simulink model "TRAS_identification"  (R2013a)
settings: Solver=ode5  SolverMode=SingleTasking  StartTime=0.0  StopTime=stop_time  FixedStep=sampling_time  RelTol=1e-3  AbsTol=1e-6
undefined symbols (not defined in the file): rtdac4pcibaseaddress
libraries: simulink x2
settings Model: SimulationMode=external  ExtModeTrigDuration=12000  ExtModeTrigLevel=0.400000  Creator=jims  LastModifiedBy=calc2
settings DataIOCC: ExternalInput=[]  InitialState=[]  LimitDataPoints=off  MaxDataPoints=5000  SignalLoggingSaveFormat=ModelDataLogs  SaveOutput=off  SaveTime=off  SignalLoggingName=sigsOut
settings OptimizationCC: BooleanDataType=off  ExpressionDepthLimit=2147483647  InitFltsAndDblsToZero=on
settings DebuggingCC: SaveWithParameterizedLinksMsg=none  MergeDetectMultiDrivingBlocksExec=error  SolverPrmCheckMsg=none  MultiTaskDSMMsg=warning  MultiTaskCondExecSysMsg=none  IntegerOverflowMsg=none  FcnCallInpInsideContextMsg=EnableAllAsWarning  StrictBusMsg=None
settings HardwareCC: TargetEndianess=LittleEndian  TargetHWDeviceType=MATLAB Host
settings RTWCC: SystemTargetFile=rtwin.tlc  TemplateMakefile=rtwin.tmf  Description=Real-Time Windows Target  ProcessScript=rtwin_make_rtw_hook  IncludeERTFirstTime=on
settings RTWinTargetCC: TargetFcnLib=ansi_tfl_tmw.mat  TargetLibSuffix=_rtwin.lib  TargetPreCompLibLocation=C:\Program Files\MATLAB\R2013a\toolbox\rtw\targets\rtwin\lib\win32  CodeReplacementLibrary=ANSI_C  ModelReferenceCompliant=off  CompOptLevelCompliant=off  RTWinDir=C:/PROGRA~1/MATLAB/R2013a/toolbox/rtw/targets/rtwin  TargetArch=win32

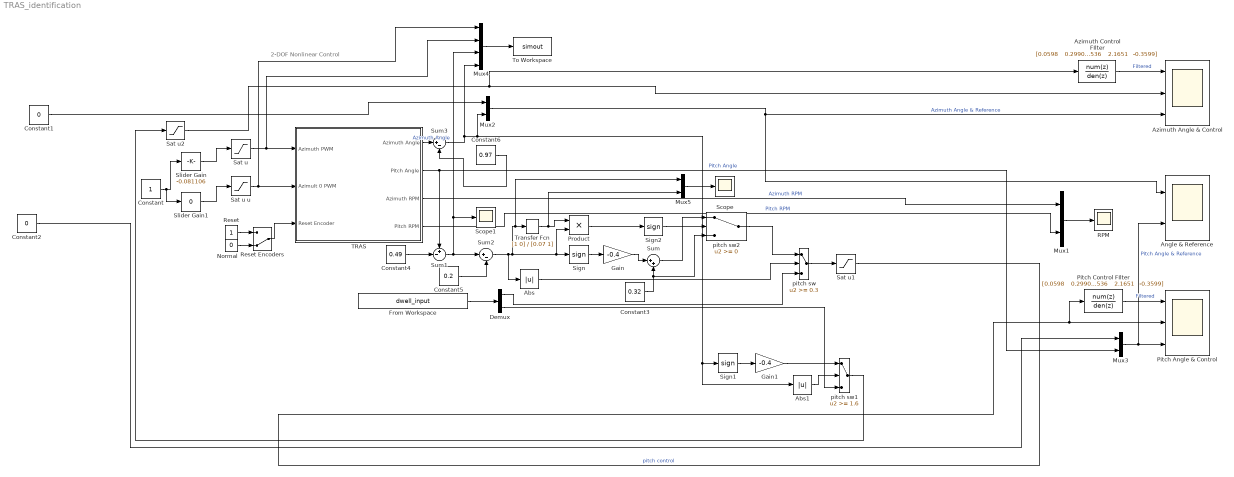
== system TRAS_identification ==
  note: 2-DOF Nonlinear Control
  Abs : Abs
  Abs1 : Abs
  Angle & Reference : Scope  NumInputPorts=2
      settings: TimeRange=90  YMin=-1~-0.5  YMax=1~0.4  SaveName=AngleReference_  MaxDataPoints=12000
  Azimuth Angle & Control : Scope  NumInputPorts=3
      settings: TimeRange=90  YMin=-0.4~-0.5~-1  YMax=-0.225~0.5~1  SaveName=AngleCtrl_  MaxDataPoints=12000
  Azimuth Control FIlter : DiscreteTransferFcn  Numerator="[0.0598    0.2990    0.5980    0.5980    0.2990    0.0598] * 1e-3"  Denominator="[1.0000   -3.9845    6.4349   -5.2536    2.1651   -0.3599]"  SampleTime=0.01
  Constant : Constant
  Constant1 : Constant  Value=0
  Constant2 : Constant  Value=0
  Constant3 : Constant  Value=0.32
  Constant4 : Constant  Value=0.49
  Constant5 : Constant  Value=0.2
  Constant6 : Constant  Value=0.97
  Demux : Demux  Outputs=2
  From Workspace : FromWorkspace  VariableName=dwell_input
  Gain : Gain  Gain=-0.4
  Gain1 : Gain  Gain=-0.4
  Mux{1..3,5} (4 alike) : Mux  Inputs=2
  Mux4 : Mux
  Normal : Constant  Value=0
  Pitch Angle & Control : Scope  NumInputPorts=3
      settings: TimeRange=90  YMin=2.77556e-17~-0.1~-0.5  YMax=0.75~0.9~0.35  SaveName=AngleCtrl1_  MaxDataPoints=12000
  Pitch Control FIlter : DiscreteTransferFcn  Numerator="[0.0598    0.2990    0.5980    0.5980    0.2990    0.0598] * 1e-3"  Denominator="[1.0000   -3.9845    6.4349   -5.2536    2.1651   -0.3599]"  SampleTime=0.01
  Product : Product
  RPM : Scope
      settings: TimeRange=90  YMin=-6000  YMax=7000  SaveName=RPM_  MaxDataPoints=12000
  Reset : Constant
  Reset Encoders : ManualSwitch  CurrentSetting=0
  Sat u : Saturate  UpperLimit=1  LowerLimit=-1
  Sat u u : Saturate  UpperLimit=1  LowerLimit=-1
  Sat u1 : Saturate  UpperLimit=1  LowerLimit=-1
  Sat u2 : Saturate  UpperLimit=1  LowerLimit=-1
  Scope : Scope
      settings: YMin=-2  YMax=2.25
  Scope1 : Scope
  Sign : Signum
  Sign1 : Signum
  Sign2 : Signum
  Slider Gain : simulink/Math Operations/Slider Gain  low=-1  gain=-0.081106  high=1
  Slider Gain1 : simulink/Math Operations/Slider Gain  low=-1  gain=0  high=1
  Sum : Sum  Inputs=|++
  Sum1 : Sum  Inputs=+-|
  Sum2 : Sum  Inputs=|+-
  Sum3 : Sum  Inputs=|+-
  TRAS : Subsystem  mask{BaseAddress=rtdac4pcibaseaddress, T0=0.01}
      mask prompts: BaseAddress "Base Address:"; T0 "Sampling Period:"
      mask Display: image(imread('TRAS.JPG'))
  To Workspace : ToWorkspace  VariableName=simout  SampleTime=-1  SaveFormat=Structure With Time
  Transfer Fcn : TransferFcn  Numerator=[1 0]  Denominator=[0.07 1]
  pitch sw : Switch  Threshold=0.3
  pitch sw1 : Switch  Threshold=1.6
  pitch sw2 : Switch
  wires:
  Pitch Control FIlter/1 -> Pitch Angle & Control/1  "Filtered"
  Mux3/1 -> Pitch Angle & Control/3, Angle & Reference/2  "Pitch Angle & Reference"
  TRAS/2(Pitch Angle) -> Sum1/1, Mux3/2  "Pitch Angle"
  Mux1/1 -> RPM/1
  Sat u2/1 -> Azimuth Angle & Control/2, Azimuth Control FIlter/1
  Sat u1/1 -> Pitch Angle & Control/2, Pitch Control FIlter/1  "pitch control"
  Azimuth Control FIlter/1 -> Azimuth Angle & Control/1  "Filtered"
  Mux2/1 -> Azimuth Angle & Control/3, Angle & Reference/1  "Azimuth Angle & Reference"
  Reset Encoders/1 -> TRAS/3(Reset Encoder)
  Reset/1 -> Reset Encoders/1
  Normal/1 -> Reset Encoders/2
  TRAS/4(Pitch RPM) -> Mux1/2  "Pitch RPM"
  TRAS/3(Azimuth RPM) -> Mux1/1  "Azimuth RPM"
  TRAS/1(Azimuth Angle) -> Sum3/1  "Azimuth Angle"
  Constant1/1 -> Mux2/1
  Constant2/1 -> Mux3/1
  From Workspace/1 -> Demux/1
  Mux4/1 -> To Workspace/1
  Sign/1 -> Gain/1
  Sum1/1 -> Scope1/1, Mux4/3, Sum2/1
  Constant4/1 -> Sum1/2
  Abs/1 -> pitch sw/2
  Demux/1 -> pitch sw/3
  pitch sw/1 -> Sat u1/1
  Gain1/1 -> pitch sw1/1
  Sign1/1 -> Gain1/1
  Abs1/1 -> pitch sw1/2
  Demux/2 -> pitch sw1/3
  pitch sw1/1 -> Sat u2/1
  Constant5/1 -> Sum2/2
  Sum2/1 -> Abs/1, Mux5/1, Transfer Fcn/1, Product/2, Sign/1
  Sum3/1 -> Mux4/4, Mux2/2, Abs1/1, Sign1/1
  Constant6/1 -> Sum3/2
  Product/1 -> Sign2/1
  Transfer Fcn/1 -> Mux5/2, Product/1
  Sign2/1 -> pitch sw2/2
  Gain/1 -> Sum/1
  Constant3/1 -> pitch sw2/3, Sum/2
  Sum/1 -> pitch sw2/1
  pitch sw2/1 -> pitch sw/1
  Mux5/1 -> Scope/1
  Sat u/1 -> Mux4/2, TRAS/1(Azimuth PWM)
  Sat u u/1 -> Mux4/1, TRAS/2(Azimult 0 PWM)
  Constant/1 -> Slider Gain1/1, Slider Gain/1
  Slider Gain/1 -> Sat u/1
  Slider Gain1/1 -> Sat u u/1

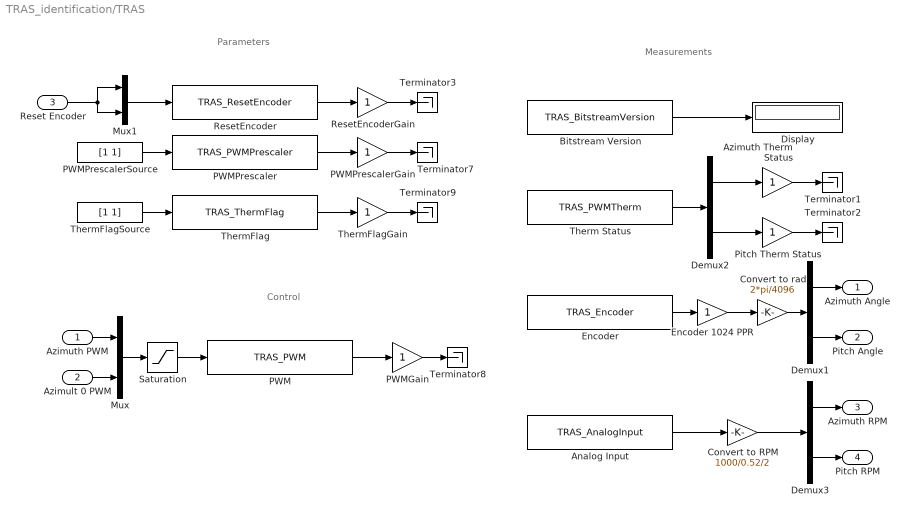
== system TRAS_identification/TRAS ==
  note: Parameters
  note: Control
  note: Measurements
  Azimuth PWM : Inport
  Azimult 0 PWM : Inport  Port=2
  Reset Encoder : Inport  Port=3
  Analog Input : S-Function  FunctionName=TRAS_AnalogInput  Parameters=BaseAddress, [1 0], [1 1], T0  EnableBusSupport=off
  Azimuth Therm Status : Gain  SaturateOnIntegerOverflow=on  OutDataTypeStr=Inherit: Same as input  ParamDataTypeStr=Inherit: Same as input
  Bitstream Version : S-Function  FunctionName=TRAS_BitstreamVersion  Parameters=BaseAddress, T0  EnableBusSupport=off
  Convert to RPM : Gain  Gain=1000/0.52/2  SaturateOnIntegerOverflow=on  OutDataTypeStr=Inherit: Same as input  ParamDataTypeStr=Inherit: Same as input
  Convert to rad : Gain  Gain=2*pi/4096  SaturateOnIntegerOverflow=on  OutDataTypeStr=Inherit: Same as input  ParamDataTypeStr=Inherit: Same as input
  Demux1 : Demux  Outputs=2
  Demux2 : Demux  Outputs=2
  Demux3 : Demux  Outputs=2
  Display : Display
  Encoder : S-Function  FunctionName=TRAS_Encoder  Parameters=BaseAddress, T0  EnableBusSupport=off
  Encoder 1024 PPR : Gain  SaturateOnIntegerOverflow=on  OutDataTypeStr=Inherit: Same as input  ParamDataTypeStr=Inherit: Same as input
  Mux : Mux  Inputs=2
  Mux1 : Mux  Inputs=2
  PWM : S-Function  FunctionName=TRAS_PWM  Parameters=BaseAddress, T0  EnableBusSupport=off
  PWMGain : Gain  SaturateOnIntegerOverflow=on  OutDataTypeStr=Inherit: Same as input  ParamDataTypeStr=Inherit: Same as input
  PWMPrescaler : S-Function  FunctionName=TRAS_PWMPrescaler  Parameters=BaseAddress, T0  EnableBusSupport=off
  PWMPrescalerGain : Gain  SaturateOnIntegerOverflow=on  OutDataTypeStr=Inherit: Same as input  ParamDataTypeStr=Inherit: Same as input
  PWMPrescalerSource : Constant  Value=[1 1]
  Pitch Therm Status : Gain  SaturateOnIntegerOverflow=on  OutDataTypeStr=Inherit: Same as input  ParamDataTypeStr=Inherit: Same as input
  ResetEncoder : S-Function  FunctionName=TRAS_ResetEncoder  Parameters=BaseAddress, T0  EnableBusSupport=off
  ResetEncoderGain : Gain  SaturateOnIntegerOverflow=on  OutDataTypeStr=Inherit: Same as input  ParamDataTypeStr=Inherit: Same as input
  Saturation : Saturate  UpperLimit=1  LowerLimit=-1
  Terminator{1..3,7..9} (6 alike) : Terminator
  Therm Status : S-Function  FunctionName=TRAS_PWMTherm  Parameters=BaseAddress, T0  EnableBusSupport=off
  "ThermFlag " : S-Function  FunctionName=TRAS_ThermFlag  Parameters=BaseAddress, T0  EnableBusSupport=off
  ThermFlagGain : Gain  SaturateOnIntegerOverflow=on  OutDataTypeStr=Inherit: Same as input  ParamDataTypeStr=Inherit: Same as input
  ThermFlagSource : Constant  Value=[1 1]
  Azimuth Angle : Outport  InitialOutput=0
  Pitch Angle : Outport  Port=2  InitialOutput=0
  Azimuth RPM : Outport  Port=3  InitialOutput=0
  Pitch RPM : Outport  Port=4  InitialOutput=0
  wires:
  Encoder 1024 PPR/1 -> Convert to rad/1
  Encoder/1 -> Encoder 1024 PPR/1
  Saturation/1 -> PWM/1
  Mux/1 -> Saturation/1
  PWM/1 -> PWMGain/1
  PWMGain/1 -> Terminator8/1
  ResetEncoder/1 -> ResetEncoderGain/1
  PWMPrescaler/1 -> PWMPrescalerGain/1
  Mux1/1 -> ResetEncoder/1
  PWMPrescalerSource/1 -> PWMPrescaler/1
  ResetEncoderGain/1 -> Terminator3/1
  PWMPrescalerGain/1 -> Terminator7/1
  Azimult 0 PWM/1 -> Mux/2
  Azimuth PWM/1 -> Mux/1
  Demux1/2 -> Pitch Angle/1
  Convert to rad/1 -> Demux1/1
  Demux1/1 -> Azimuth Angle/1
  Therm Status/1 -> Demux2/1
  Demux2/2 -> Pitch Therm Status/1
  Demux2/1 -> Azimuth Therm Status/1
  Azimuth Therm Status/1 -> Terminator1/1
  Pitch Therm Status/1 -> Terminator2/1
  Bitstream Version/1 -> Display/1
  Analog Input/1 -> Convert to RPM/1
  Demux3/2 -> Pitch RPM/1
  Demux3/1 -> Azimuth RPM/1
  Reset Encoder/1 -> Mux1/1, Mux1/2
  Convert to RPM/1 -> Demux3/1
  "ThermFlag "/1 -> ThermFlagGain/1
  ThermFlagSource/1 -> "ThermFlag "/1
  ThermFlagGain/1 -> Terminator9/1
